simulink subsystem "core"  (R2021b)
settings: Solver=VariableStepAuto  StartTime=0.0  StopTime=10.0  RelTol=1e-3
undefined symbols (not defined in the file): Ts, v0_ego, v0_lead, x0_ego, x0_lead
libraries: commrandsrc3 x1
settings Model: Creator=Otonom  LastModifiedBy=Otonom

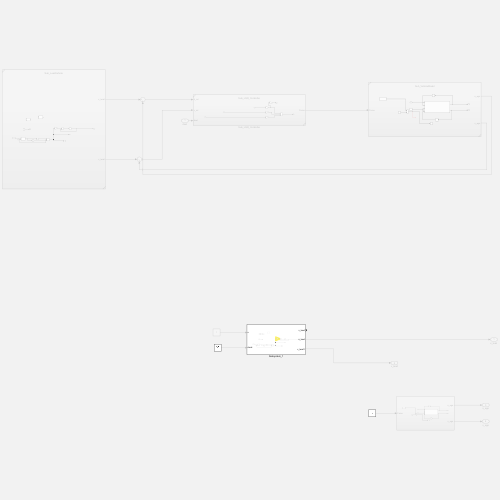
[thumbnail: Simulink's stored preview of the top-level diagram]
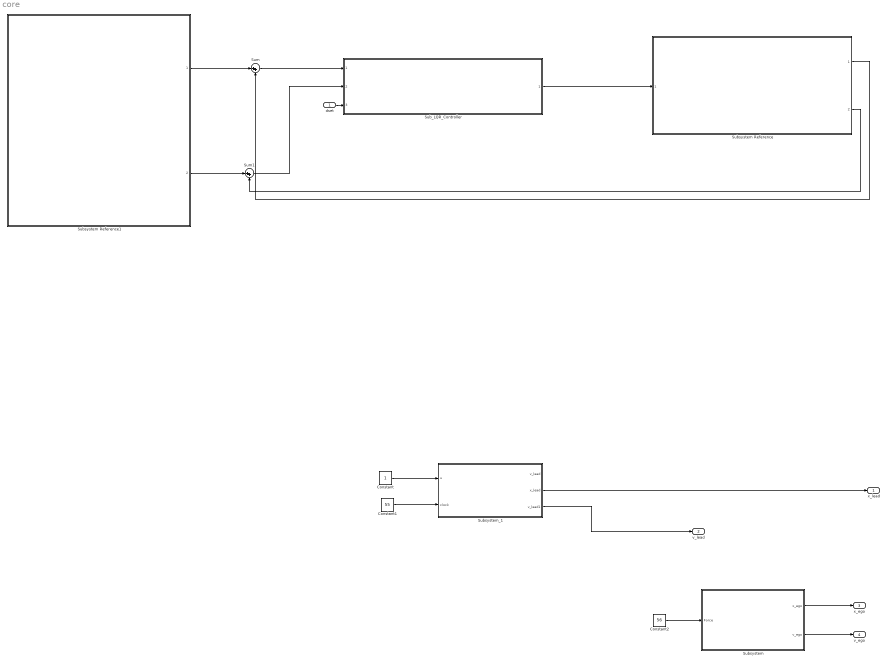
== system core ==
  dset : Inport
  Constant : Constant
  Constant1 : Constant  Value=55
  Constant2 : Constant  Value=56
  Sub_LQR_Controller : Subsystem  ReferencedSubsystem=Sub_LQR_Controller
  Subsystem : Subsystem
  Subsystem Reference : Subsystem  ReferencedSubsystem=Sub_VehicleModel
  Subsystem Reference1 : Subsystem  ReferencedSubsystem=Sub_LeadVehicle
  Subsystem_1 : Subsystem
  Sum : Sum  Inputs=|++
  Sum1 : Sum  Inputs=|++
  x_lead : Outport
  v_lead : Outport  Port=2
  x_ego : Outport  Port=3
  v_ego : Outport  Port=4
  wires:
  dset/1 -> Sub_LQR_Controller/3
  Sum/1 -> Sub_LQR_Controller/1
  Subsystem Reference/1 -> Sum/2
  Sum1/1 -> Sub_LQR_Controller/2
  Subsystem Reference1/1 -> Sum/1
  Subsystem Reference/2 -> Sum1/2
  Sub_LQR_Controller/1 -> Subsystem Reference/1
  Subsystem Reference1/2 -> Sum1/1
  Subsystem_1/2(x_lead) -> x_lead/1
  Subsystem_1/3(v_lead1) -> v_lead/1
  Constant2/1 -> Subsystem/1(Force)
  Subsystem/1(x_ego) -> x_ego/1
  Subsystem/2(v_ego) -> v_ego/1
  Constant/1 -> Subsystem_1/1(u)
  Constant1/1 -> Subsystem_1/2(clock)

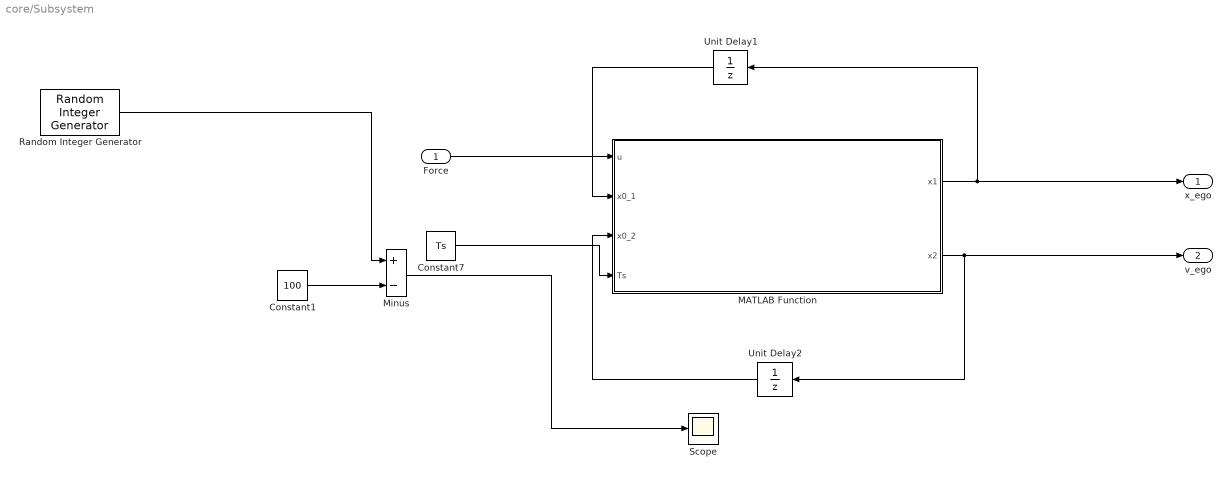
== system core/Subsystem ==
  Force : Inport
  Constant1 : Constant  Value=100
  Constant7 : Constant  Value=Ts
  MATLAB Function : MATLAB Function  TreatAsAtomicUnit=on
  Minus : Sum  Inputs=+-
  Random Integer Generator : commrandsrc3/Random Integer Generator  SetSize=150  SeedSource=Auto  Seed=0  SampleTime=0.1  SamplesPerFrame=1  OutputDataType=double  SimulateUsing=Interpreted execution
  Scope : Scope
  Unit Delay1 : UnitDelay  InitialCondition=x0_ego  SampleTime=-1  HasFrameUpgradeWarning=on
  Unit Delay2 : UnitDelay  InitialCondition=v0_ego  SampleTime=-1  HasFrameUpgradeWarning=on
  x_ego : Outport
  v_ego : Outport  Port=2
  wires:
  MATLAB Function/2(x2) -> v_ego/1, Unit Delay2/1
  Random Integer Generator/1 -> Minus/1
  MATLAB Function/1(x1) -> x_ego/1, Unit Delay1/1
  Unit Delay2/1 -> MATLAB Function/3(x0_2)
  Constant7/1 -> MATLAB Function/4(Ts)
  Minus/1 -> Scope/1
  Unit Delay1/1 -> MATLAB Function/2(x0_1)
  Force/1 -> MATLAB Function/1(u)
  Constant1/1 -> Minus/2

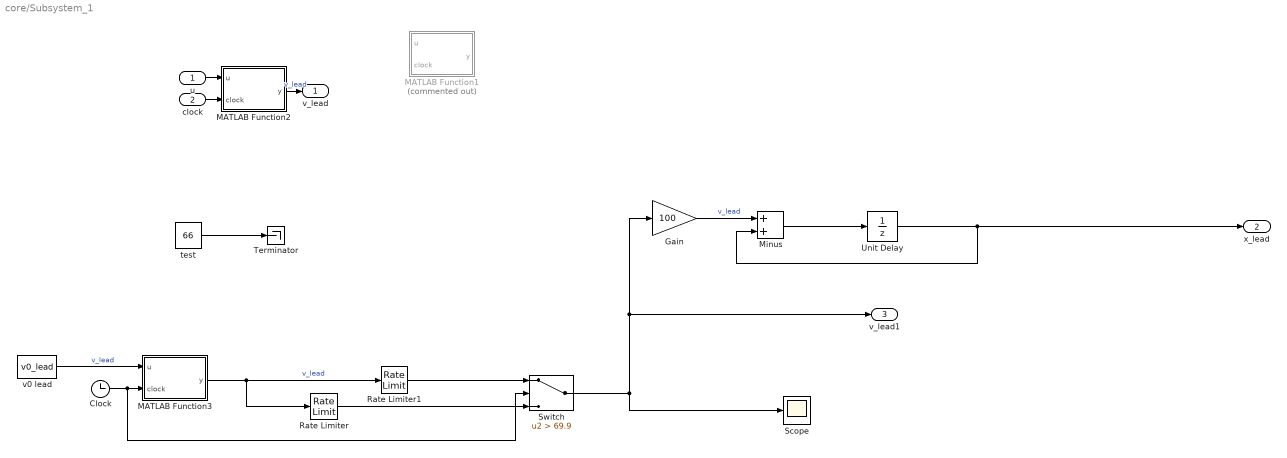
== system core/Subsystem_1 ==
  u : Inport
  clock : Inport  Port=2
  Clock : Clock
  Gain : Gain  Gain=100
  MATLAB Function1 : MATLAB Function  Commented=on  TreatAsAtomicUnit=on
  MATLAB Function2 : MATLAB Function  TreatAsAtomicUnit=on
  MATLAB Function3 : MATLAB Function  TreatAsAtomicUnit=on
  Minus : Sum
  Rate Limiter : RateLimiter  RisingSlewLimit=0.3  FallingSlewLimit=-0.3  SampleTimeMode=inherited
  Rate Limiter1 : RateLimiter  RisingSlewLimit=5  FallingSlewLimit=-5  SampleTimeMode=inherited
  Scope : Scope
  Switch : Switch  Criteria=u2 > Threshold  Threshold=69.9
  Terminator : Terminator
  Unit Delay : UnitDelay  InitialCondition=x0_lead  SampleTime=-1  HasFrameUpgradeWarning=on
  test : Constant  Value=66
  v0 lead : Constant  Value=v0_lead  SampleTime=-1
  v_lead : Outport
  x_lead : Outport  Port=2
  v_lead1 : Outport  Port=3
  wires:
  Rate Limiter1/1 -> Switch/1
  v0 lead/1 -> MATLAB Function3/1(u)  "v_lead"
  MATLAB Function3/1(y) -> Rate Limiter/1, Rate Limiter1/1  "v_lead"
  Unit Delay/1 -> x_lead/1, Minus/2
  Clock/1 -> MATLAB Function3/2(clock), Switch/2
  Minus/1 -> Unit Delay/1
  Gain/1 -> Minus/1  "v_lead"
  Rate Limiter/1 -> Switch/3
  Switch/1 -> v_lead1/1, Gain/1, Scope/1
  test/1 -> Terminator/1
  u/1 -> MATLAB Function2/1(u)
  MATLAB Function2/1(y) -> v_lead/1  "v_lead"
  clock/1 -> MATLAB Function2/2(clock)

== matlab function core/Subsystem_1/MATLAB Function1 ==
  data: u input; y output; clock input
function y = fcn(u, clock)
    if clock > 30 && clock<70
        y=u+1;
    elseif clock > 70 
        y=0;        
    else
        y=u;
    end

end

== matlab function core/Subsystem_1/MATLAB Function2 ==
  data: u input; y output; clock input
function y = fcn(u, clock)
    if clock > 30 
        y=0;
    else
        y=u;
    end
    

end

== matlab function core/Subsystem_1/MATLAB Function3 ==
  data: u input; y output; clock input
function y = fcn(u, clock)
    if clock > 30 && clock<70
        y=u+3;
    elseif clock > 70 
        y=2;        
    else
        y=u;
    end

end

== matlab function core/Subsystem/MATLAB Function ==
  data: u input; x1 output; x0_1 input; x0_2 input; x2 output; Ts input
function [x1, x2] = fcn(u, x0_1, x0_2, Ts)
    m = 4700;
    b = 444;
    delta = Ts;

    A_init = [0 1.0000; 0 -b/m];
    B_init = [0; 1/m];

    A = A_init * delta + eye(2);
    B = B_init * delta;
    C = [1 0];

    x0 = [x0_1; x0_2];
    y = A * x0 + B * u;

    x1 = y(1);
    x2 = y(2);
end
